simulink model "P2Q5"  (R2018a)
settings: Solver=VariableStepAuto  StartTime=0.0  StopTime=0.3  RelTol=1e-3
libraries: dspstat3 x3, dspmathops x3, dsparch4 x2, dspsrcs4 x1, simulink x1
settings Model: Creator=Marine  LastModifiedBy=ifaruk

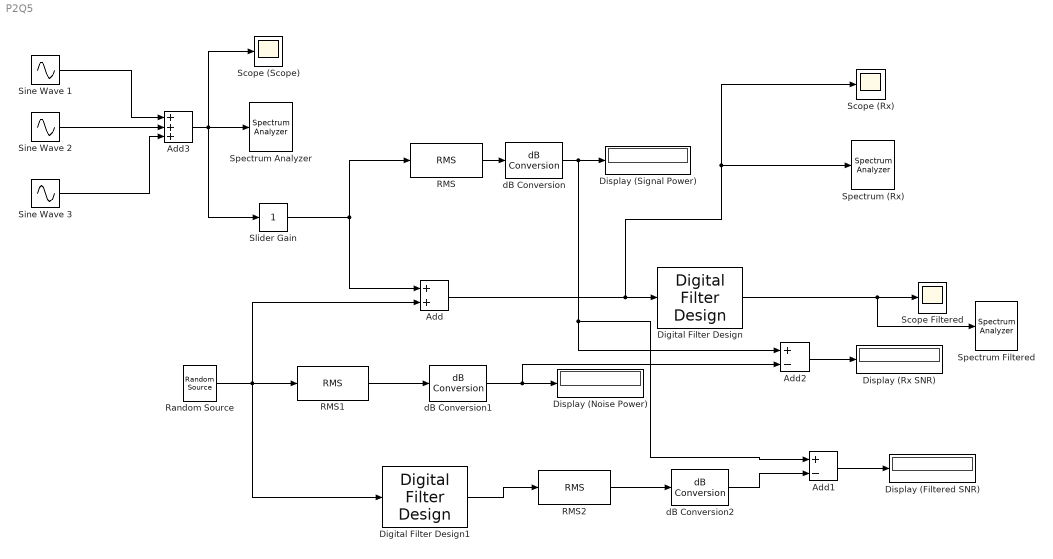
== system P2Q5 ==
  Add : Sum
  Add1 : Sum  Inputs=+-
  Add2 : Sum  Inputs=+-
  Add3 : Sum  Inputs=+++
  Digital Filter Design : dsparch4/Digital Filter Design  mwdsp_browser_bugfix_var=off
  Digital Filter Design1 : dsparch4/Digital Filter Design  mwdsp_browser_bugfix_var=off
  Display (Filtered SNR) : Display
  Display (Noise Power) : Display
  Display (Rx SNR) : Display
  Display (Signal Power) : Display
  RMS : dspstat3/RMS  run=on  directionMode=Each column  dimension=1  InputProcessing=Columns as channels (frame based)  reset_popup=None
  RMS1 : dspstat3/RMS  run=on  directionMode=Each column  dimension=1  InputProcessing=Columns as channels (frame based)  reset_popup=None
  RMS2 : dspstat3/RMS  run=on  directionMode=Each column  dimension=1  InputProcessing=Columns as channels (frame based)  reset_popup=None
  Random Source : dspsrcs4/Random Source  SrcType=Gaussian  NormMethod=Ziggurat  CltLength=12  MinVal=0  MaxVal=1  MeanVal=0  VarVal=1  RepMode=Not repeatable  rawSeed=1  IsInherit=off  SampMode=Discrete  SampTime=0.0001  SampFrame=1  DataType=Double  OutComplex=Real  OutputFrames=off
  Scope (Rx) : Scope
  Scope (Scope) : Scope
  Scope Filtered : Scope
  Sine Wave 1 : Sin  SineType=Sample based  Amplitude=0.5  Samples=1000  SampleTime=0.0001
  "Sine Wave 2 " : Sin  SineType=Sample based  Amplitude=2  Frequency=5000  Samples=500  SampleTime=0.0001
  "Sine Wave 3 " : Sin  SineType=Sample based  Amplitude=1.5  Samples=100  SampleTime=0.0001
  Slider Gain : simulink/Math Operations/Slider Gain  gain=1  low=0  high=12
  Spectrum (Rx) : SpectrumAnalyzer
  Spectrum Analyzer : SpectrumAnalyzer
  Spectrum Filtered : SpectrumAnalyzer
  dB Conversion : dspmathops/dB Conversion  dBtype=dB  intype=Amplitude  R=1  fuzz=off
      settings: SourceProductName=DSP System Toolbox
  dB Conversion1 : dspmathops/dB Conversion  dBtype=dB  intype=Amplitude  R=1  fuzz=off
      settings: SourceProductName=DSP System Toolbox
  dB Conversion2 : dspmathops/dB Conversion  dBtype=dB  intype=Amplitude  R=1  fuzz=off
      settings: SourceProductName=DSP System Toolbox
  wires:
  Add3/1 -> Slider Gain/1, Spectrum Analyzer/1, Scope (Scope)/1
  Slider Gain/1 -> Add/1, RMS/1
  RMS/1 -> dB Conversion/1
  dB Conversion/1 -> Add1/1, Add2/1, Display (Signal Power)/1
  Random Source/1 -> Add/2, Digital Filter Design1/1, RMS1/1
  RMS1/1 -> dB Conversion1/1
  dB Conversion1/1 -> Add2/2, Display (Noise Power)/1
  Digital Filter Design1/1 -> RMS2/1
  RMS2/1 -> dB Conversion2/1
  Add1/1 -> Display (Filtered SNR)/1
  dB Conversion2/1 -> Add1/2
  Add/1 -> Scope (Rx)/1, Spectrum (Rx)/1, Digital Filter Design/1
  Digital Filter Design/1 -> Spectrum Filtered/1, Scope Filtered/1
  Add2/1 -> Display (Rx SNR)/1
  "Sine Wave 2 "/1 -> Add3/2
  "Sine Wave 3 "/1 -> Add3/3
  Sine Wave 1/1 -> Add3/1
